simulink model "Verificacion_planta"  (R2021a)
settings: Solver=ode45  StartTime=0.0  StopTime=1000  MaxStep=0.1  RelTol=1e-6  EnableMultiTasking=on
values from neighbouring files (symbols this model uses):
  den = [tau 1]    [TP1resolucion.m]
  num = [k]    [TP1resolucion.m]
undefined symbols (not defined in the file or in its folder): Ce0, Fh0
settings Model: Creator=Marcelo  LastModifiedBy=Fer
settings SolverCC: AlgebraicLoopSolver=TrustRegion
settings DataIOCC: SaveFormat=Array  SignalLoggingSaveFormat=ModelDataLogs  SaveOutput=off  ReturnWorkspaceOutputs=off  SignalLoggingName=sigsOut
settings OptimizationCC: BlockReduction=off  BooleanDataType=off  ExpressionDepthLimit=2147483647  LifeSpan=inf
settings DebuggingCC: SaveWithParameterizedLinksMsg=none  UnderspecifiedInitializationDetection=Classic  MergeDetectMultiDrivingBlocksExec=none  SignalResolutionControl=TryResolveAllWithWarning  MultiTaskDSMMsg=warning  MultiTaskCondExecSysMsg=none  FcnCallInpInsideContextMsg=warning  StateNameClashWarn=warning  SFUnexpectedBacktrackingDiag=warning  SFNoUnconditionalDefaultTransitionDiag=warning  SFExecutionAtInitializationDiag=none  SFMachineParentedDataDiag=warning  ArithmeticOperatorsInVariantConditions=warning
settings HardwareCC: ProdBitPerPointer=32  ProdBitPerSizeT=32  ProdBitPerPtrDiffT=32  ProdLargestAtomicFloat=None  ProdIntDivRoundTo=Undefined  ProdEndianess=Unspecified  ProdWordSize=32  ProdHWDeviceType=32-bit Generic  TargetUnknown=on
settings ModelReferenceCC: PropagateSignalLabelsOutOfModel=off
settings SFSimCC: SimUseLocalCustomCode=off  CustomCodeUndefinedFunction=UseInterfaceOnly
settings RTWCC: RTWUseLocalCustomCode=off
settings CodeAppCC: StateflowObjectComments=on
settings GRTTargetCC: TargetLangStandard=C89/C90 (ANSI)  CombineOutputUpdateFcns=off  GRTInterface=on
settings ConfigComp: CovMetricSettings=dw  CovSaveCumulativeToWorkspaceVar=on  CovSaveSingleToWorkspaceVar=on  CovExternalEMLEnable=off

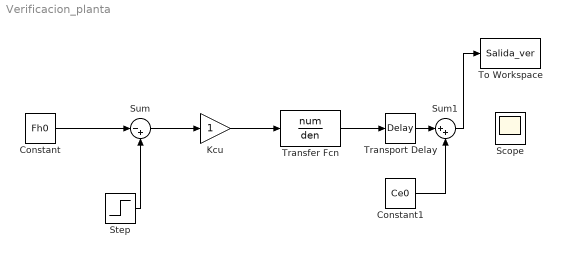
== system Verificacion_planta ==
  Constant : Constant  Value=Fh0
  Constant1 : Constant  Value=Ce0
  Kcu : Gain
  Scope : Scope
  Step : Step  Time=100  Before=Fh0  After=Fh0*1.04  SampleTime=0
  Sum : Sum  Inputs=|-+
  Sum1 : Sum  Inputs=|++
  To Workspace : ToWorkspace  VariableName=Salida_ver
  Transfer Fcn : TransferFcn  Numerator=num  Denominator=den
  Transport Delay : TransportDelay  DelayTime=21.3
  wires:
  Transfer Fcn/1 -> Transport Delay/1
  Kcu/1 -> Transfer Fcn/1
  Step/1 -> Sum/2
  Sum/1 -> Kcu/1
  Constant/1 -> Sum/1
  Transport Delay/1 -> Sum1/1
  Constant1/1 -> Sum1/2
  Sum1/1 -> To Workspace/1
